simulink model "fd_scheme"  (R2022a)
settings: Solver=VariableStepAuto  StartTime=0.0  StopTime=10.0  RelTol=1e-3
undefined symbols (not defined in the file or in its folder): q_dot_0
settings Model: Creator=charl  LastModifiedBy=charl

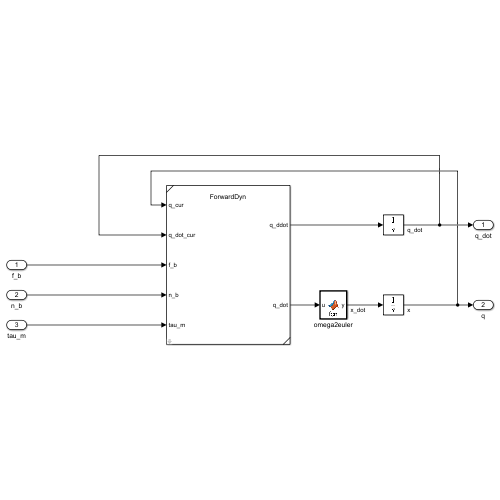
[thumbnail: Simulink's stored preview of the top-level diagram]
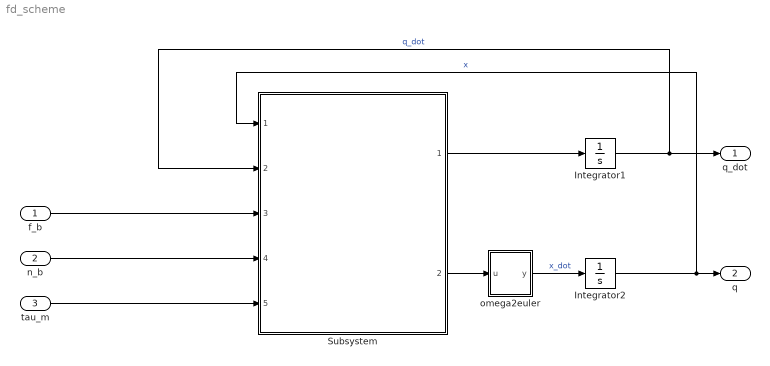
== system fd_scheme ==
  f_b : Inport
  n_b : Inport  Port=2
  tau_m : Inport  Port=3
  Integrator1 : Integrator  InitialCondition=q_dot_0
  Integrator2 : Integrator
  Subsystem : Subsystem  ReferencedSubsystem=ForwardDyn
  omega2euler : MATLAB Function  TreatAsAtomicUnit=on
  q_dot : Outport
  q : Outport  Port=2
  wires:
  Subsystem/1 -> Integrator1/1
  Integrator1/1 -> Subsystem/2, q_dot/1  "q_dot"
  omega2euler/1(y) -> Integrator2/1  "x_dot"
  Integrator2/1 -> Subsystem/1, q/1  "x"
  f_b/1 -> Subsystem/3
  n_b/1 -> Subsystem/4
  tau_m/1 -> Subsystem/5
  Subsystem/2 -> omega2euler/1(u)

== matlab function fd_scheme/omega2euler ==
  data: u input; y output
function y = fcn(u)

y = u;
